simulink model "Question_1_Sim"  (R2022b)
settings: Solver=VariableStepAuto  StartTime=0.0  StopTime=10.0  RelTol=1e-3
values from neighbouring files (symbols this model uses):
  b1 = 40    [Question_1_mat.m]    (also in question_3_mat.m = 36)
  b2 = 30    [Question_1_mat.m]    (also in question_3_mat.m = 26)
  g = 9.81    [Question_1_mat.m]    (also in question_3_mat.m)
  k = 5    [Question_1_mat.m]    (also in question_2_mat.m = 0.2)
  m1 = 2    [Question_1_mat.m]    (also in question_2_mat.m = 1; question_3_mat.m)
  m2 = 3    [Question_1_mat.m]    (also in question_2_mat.m = 1.5; question_3_mat.m)
  m3 = 8    [Question_1_mat.m]
settings Model: Creator=adnzw  LastModifiedBy=adnzw

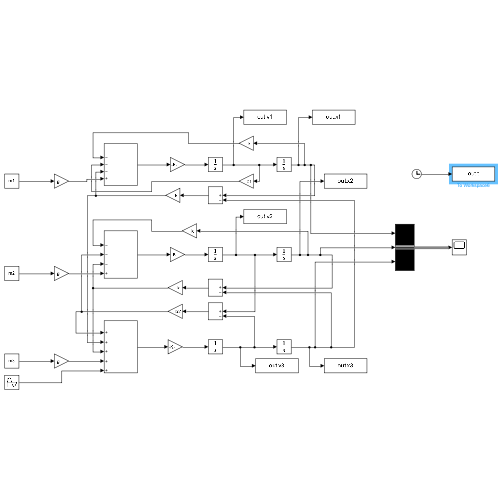
[thumbnail: Simulink's stored preview of the top-level diagram]
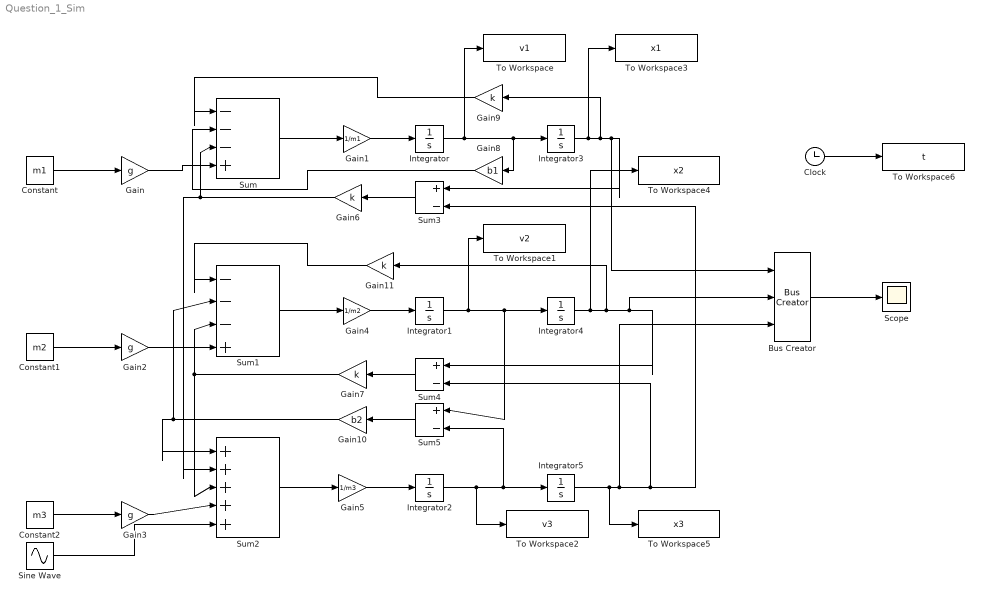
== system Question_1_Sim ==
  Bus Creator : BusCreator  Inputs=3
  Clock : Clock
  Constant : Constant  Value=m1
  Constant1 : Constant  Value=m2
  Constant2 : Constant  Value=m3
  Gain : Gain  Gain=g
  Gain1 : Gain  Gain=1/m1
  Gain10 : Gain  Gain=b2
  Gain{6..7,9,11} (4 alike) : Gain  Gain=k
  Gain2 : Gain  Gain=g
  Gain3 : Gain  Gain=g
  Gain4 : Gain  Gain=1/m2
  Gain5 : Gain  Gain=1/m3
  Gain8 : Gain  Gain=b1
  Integrator{,1..5} (6 alike) : Integrator
  Scope : Scope
  Sine Wave : Sin  SampleTime=0
  Sum : Sum  Inputs=|---+
  Sum1 : Sum  Inputs=|---+
  Sum2 : Sum  Inputs=|+++++
  Sum3 : Sum  Inputs=|+-
  Sum4 : Sum  Inputs=|+-
  Sum5 : Sum  Inputs=|+-
  To Workspace : ToWorkspace  VariableName=v1  SaveFormat=Timeseries  SampleTime=-1
  To Workspace1 : ToWorkspace  VariableName=v2  SaveFormat=Timeseries  SampleTime=-1
  To Workspace2 : ToWorkspace  VariableName=v3  SaveFormat=Timeseries  SampleTime=-1
  To Workspace3 : ToWorkspace  VariableName=x1  SaveFormat=Timeseries  SampleTime=-1
  To Workspace4 : ToWorkspace  VariableName=x2  SaveFormat=Timeseries  SampleTime=-1
  To Workspace5 : ToWorkspace  VariableName=x3  SaveFormat=Timeseries  SampleTime=-1
  To Workspace6 : ToWorkspace  VariableName=t  SaveFormat=Timeseries  SampleTime=-1
  wires:
  Constant2/1 -> Gain3/1
  Gain3/1 -> Sum2/4
  Constant1/1 -> Gain2/1
  Gain2/1 -> Sum1/4
  Constant/1 -> Gain/1
  Gain/1 -> Sum/4
  Sine Wave/1 -> Sum2/5
  Sum/1 -> Gain1/1
  Sum1/1 -> Gain4/1
  Sum2/1 -> Gain5/1
  Gain1/1 -> Integrator/1
  Integrator/1 -> To Workspace/1, Gain8/1, Integrator3/1
  Gain4/1 -> Integrator1/1
  Integrator1/1 -> To Workspace1/1, Sum5/1, Integrator4/1
  Gain5/1 -> Integrator2/1
  Integrator2/1 -> To Workspace2/1, Sum5/2, Integrator5/1
  Integrator3/1 -> To Workspace3/1, Bus Creator/1, Sum3/1, Gain9/1
  Integrator5/1 -> To Workspace5/1, Bus Creator/3, Sum4/2, Sum3/2
  Sum3/1 -> Gain6/1
  Gain6/1 -> Sum2/2, Sum/3
  Integrator4/1 -> To Workspace4/1, Gain11/1, Bus Creator/2, Sum4/1
  Sum4/1 -> Gain7/1
  Gain7/1 -> Sum2/3, Sum1/3
  Gain8/1 -> Sum/2
  Gain9/1 -> Sum/1
  Sum5/1 -> Gain10/1
  Gain10/1 -> Sum2/1, Sum1/2
  Gain11/1 -> Sum1/1
  Bus Creator/1 -> Scope/1
  Clock/1 -> To Workspace6/1
